simulink library "stand_still_Gait"  (R2024a)
settings: Solver=VariableStepAuto  StartTime=0.0  StopTime=10.0  RelTol=1e-3
undefined symbols (not defined in the file): Lower_limbs, P0x, P0z, P1x, P1z, P2x, P2z, Upper_limbs
libraries: Plane_Movement_stand_still x4
settings Model: Creator=renre  LastModifiedBy=renre

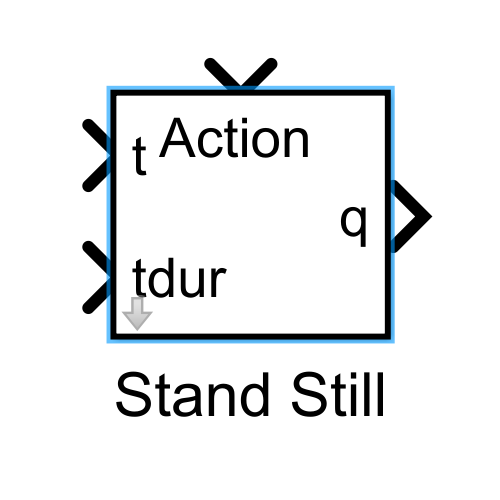
[thumbnail: Simulink's stored preview of the top-level diagram]
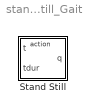
== system stand_still_Gait ==
  Stand Still : Subsystem  mask{P3x=0, P3z=-0.08}
      mask prompts: P3x "Bezier-Point 3 - X"; P3z "Bezier-Point 3- Z"

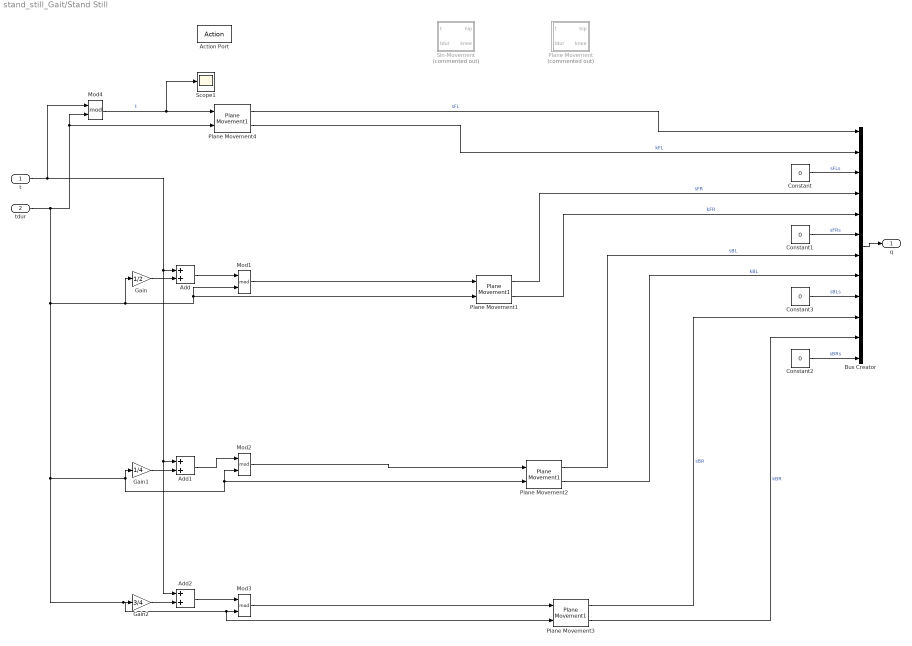
== system stand_still_Gait/Stand Still ==
  t : Inport
  tdur : Inport  Port=2
  Action Port : ActionPort  InitializeStates=reset
  Add : Sum
  Add1 : Sum
  Add2 : Sum
  Bus Creator : BusCreator  Inputs=12
  Constant{,1..3} (4 alike) : Constant  Value=0
  Gain : Gain  Gain=1/2
  Gain1 : Gain  Gain=1/4
  Gain2 : Gain  Gain=3/4
  Mod{1..4} (4 alike) : Math  Operator=mod
  Plane Movement : Subsystem  Commented=on
  Plane Movement{1..4} (4 alike) : Plane_Movement_stand_still/Plane Movement1  SystemSampleTime=-1  VariantActivationTime=update diagram  AllowFlexibleInterface=on  Latency=0  AutoFrameSizeCalculation=off
  Scope1 : Scope
  Sin-Movement : Subsystem  Commented=on
  q : Outport
  wires:
  Bus Creator/1 -> q/1
  Plane Movement4/1 -> Bus Creator/1  "sFL"
  Plane Movement1/1 -> Bus Creator/4  "sFR"
  Plane Movement4/2 -> Bus Creator/2  "kFL"
  Plane Movement1/2 -> Bus Creator/5  "kFR"
  Mod1/1 -> Plane Movement1/1
  Plane Movement2/2 -> Bus Creator/8  "kBL"
  Plane Movement2/1 -> Bus Creator/7  "sBL"
  Plane Movement3/2 -> Bus Creator/11  "kBR"
  Plane Movement3/1 -> Bus Creator/10  "sBR"
  Mod2/1 -> Plane Movement2/1
  Mod3/1 -> Plane Movement3/1
  Add/1 -> Mod1/1
  Gain/1 -> Add/2
  Add1/1 -> Mod2/1
  Gain1/1 -> Add1/2
  t/1 -> Add2/1, Add1/1, Add/1, Mod4/1
  Add2/1 -> Mod3/1
  Gain2/1 -> Add2/2
  tdur/1 -> Plane Movement4/2, Mod4/2, Gain/1, Plane Movement1/2, Mod1/2, Plane Movement3/2, Mod3/2, Gain2/1, Plane Movement2/2, Mod2/2, Gain1/1
  Mod4/1 -> Plane Movement4/1, Scope1/1  "t"
  Constant/1 -> Bus Creator/3  "sFLs"
  Constant1/1 -> Bus Creator/6  "sFRs"
  Constant3/1 -> Bus Creator/9  "sBLs"
  Constant2/1 -> Bus Creator/12  "sBRs"

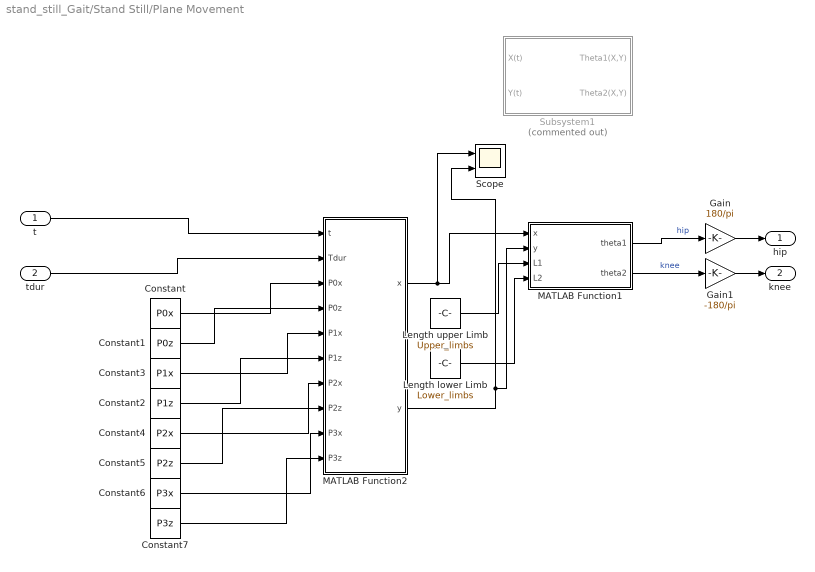
== system stand_still_Gait/Stand Still/Plane Movement ==
  t : Inport
  tdur : Inport  Port=2
  Constant : Constant  Value=P0x
  Constant1 : Constant  Value=P0z
  Constant2 : Constant  Value=P1z
  Constant3 : Constant  Value=P1x
  Constant4 : Constant  Value=P2x
  Constant5 : Constant  Value=P2z
  Constant6 : Constant  Value=P3x
  Constant7 : Constant  Value=P3z
  Gain : Gain  Gain=180/pi
  Gain1 : Gain  Gain=-180/pi
  Length lower Limb : Constant  Value=Lower_limbs
  Length upper Limb : Constant  Value=Upper_limbs
  MATLAB Function1 : MATLAB Function  TreatAsAtomicUnit=on
  MATLAB Function2 : MATLAB Function  TreatAsAtomicUnit=on
  Scope : Scope  NumInputPorts=2
  Subsystem1 : Subsystem  Commented=on
  hip : Outport
  knee : Outport  Port=2
  wires:
  MATLAB Function2/2(y) -> MATLAB Function1/2(y), Scope/2
  MATLAB Function2/1(x) -> Scope/1, MATLAB Function1/1(x)
  MATLAB Function1/2(theta2) -> Gain1/1  "knee"
  tdur/1 -> MATLAB Function2/2(Tdur)
  MATLAB Function1/1(theta1) -> Gain/1  "hip"
  t/1 -> MATLAB Function2/1(t)
  Length upper Limb/1 -> MATLAB Function1/3(L1)
  Length lower Limb/1 -> MATLAB Function1/4(L2)
  Gain1/1 -> knee/1
  Gain/1 -> hip/1
  Constant/1 -> MATLAB Function2/3(P0x)
  Constant1/1 -> MATLAB Function2/4(P0z)
  Constant3/1 -> MATLAB Function2/5(P1x)
  Constant2/1 -> MATLAB Function2/6(P1z)
  Constant4/1 -> MATLAB Function2/7(P2x)
  Constant5/1 -> MATLAB Function2/8(P2z)
  Constant6/1 -> MATLAB Function2/9(P3x)
  Constant7/1 -> MATLAB Function2/10(P3z)

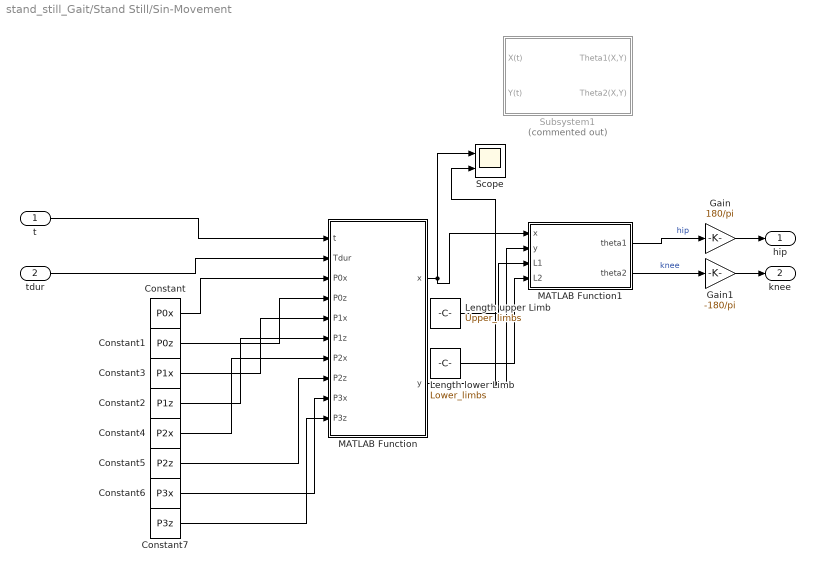
== system stand_still_Gait/Stand Still/Sin-Movement ==
  t : Inport
  tdur : Inport  Port=2
  Constant : Constant  Value=P0x
  Constant1 : Constant  Value=P0z
  Constant2 : Constant  Value=P1z
  Constant3 : Constant  Value=P1x
  Constant4 : Constant  Value=P2x
  Constant5 : Constant  Value=P2z
  Constant6 : Constant  Value=P3x
  Constant7 : Constant  Value=P3z
  Gain : Gain  Gain=180/pi
  Gain1 : Gain  Gain=-180/pi
  Length lower Limb : Constant  Value=Lower_limbs
  Length upper Limb : Constant  Value=Upper_limbs
  MATLAB Function : MATLAB Function  TreatAsAtomicUnit=on
  MATLAB Function1 : MATLAB Function  TreatAsAtomicUnit=on
  Scope : Scope  NumInputPorts=2
  Subsystem1 : Subsystem  Commented=on
  hip : Outport
  knee : Outport  Port=2
  wires:
  MATLAB Function/2(y) -> MATLAB Function1/2(y), Scope/2
  MATLAB Function/1(x) -> MATLAB Function1/1(x), Scope/1
  MATLAB Function1/2(theta2) -> Gain1/1  "knee"
  tdur/1 -> MATLAB Function/2(Tdur)
  MATLAB Function1/1(theta1) -> Gain/1  "hip"
  t/1 -> MATLAB Function/1(t)
  Length upper Limb/1 -> MATLAB Function1/3(L1)
  Length lower Limb/1 -> MATLAB Function1/4(L2)
  Gain1/1 -> knee/1
  Gain/1 -> hip/1
  Constant/1 -> MATLAB Function/3(P0x)
  Constant1/1 -> MATLAB Function/4(P0z)
  Constant3/1 -> MATLAB Function/5(P1x)
  Constant2/1 -> MATLAB Function/6(P1z)
  Constant4/1 -> MATLAB Function/7(P2x)
  Constant5/1 -> MATLAB Function/8(P2z)
  Constant6/1 -> MATLAB Function/9(P3x)
  Constant7/1 -> MATLAB Function/10(P3z)

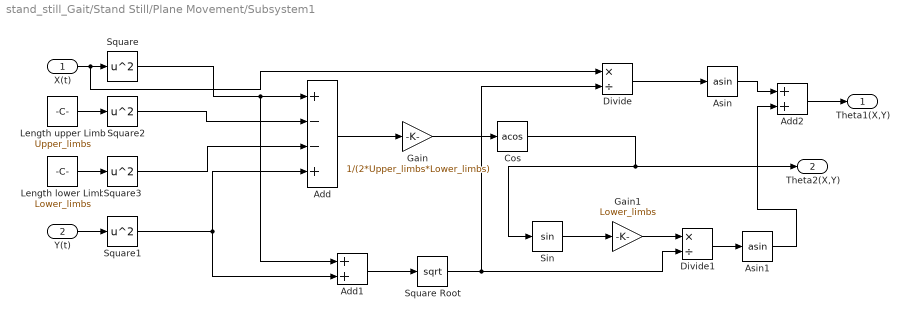
== system stand_still_Gait/Stand Still/Plane Movement/Subsystem1 ==
  X(t) : Inport
  Y(t) : Inport  Port=2
  Add : Sum  Inputs=+--+
  Add1 : Sum
  Add2 : Sum
  Asin : Trigonometry  Operator=asin
  Asin1 : Trigonometry  Operator=asin
  Cos : Trigonometry  Operator=acos
  Divide : Product  Inputs=*/
  Divide1 : Product  Inputs=*/
  Gain : Gain  Gain=1/(2*Upper_limbs*Lower_limbs)
  Gain1 : Gain  Gain=Lower_limbs
  Length lower Limb : Constant  Value=Lower_limbs
  Length upper Limb : Constant  Value=Upper_limbs
  Sin : Trigonometry
  Square{,1..3} (4 alike) : Math  Operator=square
  Square Root : Sqrt
  Theta1(X,Y) : Outport
  Theta2(X,Y) : Outport  Port=2
  wires:
  X(t)/1 -> Divide/1, Square/1
  Y(t)/1 -> Square1/1
  Square/1 -> Add1/1, Add/1
  Length upper Limb/1 -> Square2/1
  Length lower Limb/1 -> Square3/1
  Square2/1 -> Add/2
  Square3/1 -> Add/3
  Square1/1 -> Add1/2, Add/4
  Add/1 -> Gain/1
  Gain/1 -> Cos/1
  Cos/1 -> Theta2(X,Y)/1, Sin/1
  Asin/1 -> Add2/1
  Sin/1 -> Gain1/1
  Add1/1 -> Square Root/1
  Gain1/1 -> Divide1/1
  Square Root/1 -> Divide/2, Divide1/2
  Divide1/1 -> Asin1/1
  Asin1/1 -> Add2/2
  Add2/1 -> Theta1(X,Y)/1
  Divide/1 -> Asin/1

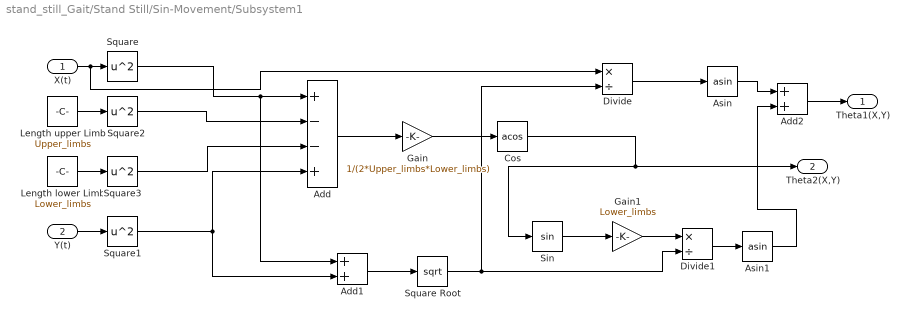
== system stand_still_Gait/Stand Still/Sin-Movement/Subsystem1 ==
  X(t) : Inport
  Y(t) : Inport  Port=2
  Add : Sum  Inputs=+--+
  Add1 : Sum
  Add2 : Sum
  Asin : Trigonometry  Operator=asin
  Asin1 : Trigonometry  Operator=asin
  Cos : Trigonometry  Operator=acos
  Divide : Product  Inputs=*/
  Divide1 : Product  Inputs=*/
  Gain : Gain  Gain=1/(2*Upper_limbs*Lower_limbs)
  Gain1 : Gain  Gain=Lower_limbs
  Length lower Limb : Constant  Value=Lower_limbs
  Length upper Limb : Constant  Value=Upper_limbs
  Sin : Trigonometry
  Square{,1..3} (4 alike) : Math  Operator=square
  Square Root : Sqrt
  Theta1(X,Y) : Outport
  Theta2(X,Y) : Outport  Port=2
  wires:
  X(t)/1 -> Divide/1, Square/1
  Y(t)/1 -> Square1/1
  Square/1 -> Add1/1, Add/1
  Length upper Limb/1 -> Square2/1
  Length lower Limb/1 -> Square3/1
  Square2/1 -> Add/2
  Square3/1 -> Add/3
  Square1/1 -> Add1/2, Add/4
  Add/1 -> Gain/1
  Gain/1 -> Cos/1
  Cos/1 -> Theta2(X,Y)/1, Sin/1
  Asin/1 -> Add2/1
  Sin/1 -> Gain1/1
  Add1/1 -> Square Root/1
  Gain1/1 -> Divide1/1
  Square Root/1 -> Divide/2, Divide1/2
  Divide1/1 -> Asin1/1
  Asin1/1 -> Add2/2
  Add2/1 -> Theta1(X,Y)/1
  Divide/1 -> Asin/1

== matlab function stand_still_Gait/Stand Still/Plane Movement/MATLAB Function1 ==
  data: x input; theta1 output; y input; L1 input; L2 input; theta2 output
function [theta1, theta2] = ang(x,y,L1,L2)
theta2 = acos((x.^2+y.^2-L1.^2-L2.^2) / (2*L1*L2));
beta = asin((L2*sin(theta2))./((x.^2+y.^2).^0.5));
theta1 = asin(x./((x.^2+y.^2).^0.5)) + beta;
end

== matlab function stand_still_Gait/Stand Still/Plane Movement/MATLAB Function2 ==
  data: x output; t input; Tdur input; y output; P0x input; P0z input; P1x input; P1z input; P2x input; P2z input; P3x input; P3z input
function [x, y] = bez_plane_TrajV2(t,Tdur,P0x,P0z,P1x,P1z,P2x,P2z,P3x,P3z)
t_swing = Tdur/4;
t_support = Tdur*3/4;

P0 = [P0x, P0z];
P1 = [P1x, P1z];
P2 = [P2x, P2z];
P3 = [P3x, P3z];
if t<=t_swing
    Sw = P0*((1-(t/t_swing))^3) + 3*P1*(t/t_swing)*((1-(t/t_swing))^2) + 3*P2*((t/t_swing)^2)*(1-(t/t_swing)) + P3*((t/t_swing)^3);
    
    x = -1*Sw(1);
    y = Sw(2);
else
    x = -1*(P3(1)+(P0(1)-P3(1))/t_support*(t-t_swing));
    y = P0(2);
end
end

== matlab function stand_still_Gait/Stand Still/Sin-Movement/MATLAB Function ==
  data: x output; t input; y output; Tdur input; P0x input; P0z input; P1x input; P1z input; P2x input; P2z input; P3x input; P3z input
function [x, y] = bezTrajV2(t, Tdur, P0x,P0z,P1x,P1z,P2x,P2z,P3x,P3z)
t_swing = Tdur/4;
t_support = Tdur*3/4;

P0 = [P0x, P0z];
P1 = [P1x, P1z];
P2 = [P2x, P2z];
P3 = [P3x, P3z];
if t<=t_swing
    Sw = P0*((1-(t/t_swing))^3) + 3*P1*(t/t_swing)*((1-(t/t_swing))^2) + 3*P2*((t/t_swing)^2)*(1-(t/t_swing)) + P3*((t/t_swing)^3);
    
    x = -1*Sw(1);
    y = Sw(2);
else
    x = -1*(P3(1)+(P0(1)-P3(1))/t_support*(t-t_swing));
    y = -0.003*sin((x-P0(1))*pi/(P3(1)-P0(1)))+P0(2);
end
end

== matlab function stand_still_Gait/Stand Still/Sin-Movement/MATLAB Function1 ==
  data: x input; theta1 output; y input; L1 input; L2 input; theta2 output
function [theta1, theta2] = ang(x,y,L1,L2)
theta2 = acos((x.^2+y.^2-L1.^2-L2.^2) / (2*L1*L2));
beta = asin((L2*sin(theta2))./((x.^2+y.^2).^0.5));
theta1 = asin(x./((x.^2+y.^2).^0.5)) + beta;
end
